simulink model "task8b_v23"  (R2023b)
settings: Solver=VariableStepAuto  StartTime=0.0  StopTime=10.0  RelTol=1e-3
values from neighbouring files (symbols this model uses):
  tInterval = [0 5]    [task7b2.m]    (also in task8b_setup.m = [0 10]; task9_visu.m = [0 10]; task9b_setup.m = [0 10])
undefined symbols (not defined in the file or in its folder): eul2tform, trvec2tform
libraries: robotcorelib x5, robotmaniplib x1
settings Model: Creator=Nico  LastModifiedBy=Nico
settings DebuggingCC: UnderSpecifiedDimensionMsg=warning
settings RTWCC: GPUComputeCapability=5.0

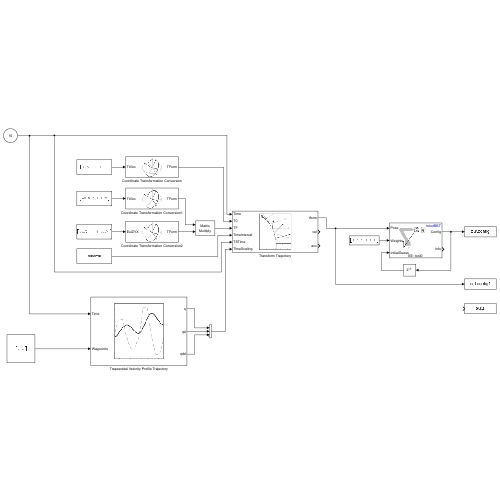
[thumbnail: Simulink's stored preview of the top-level diagram]
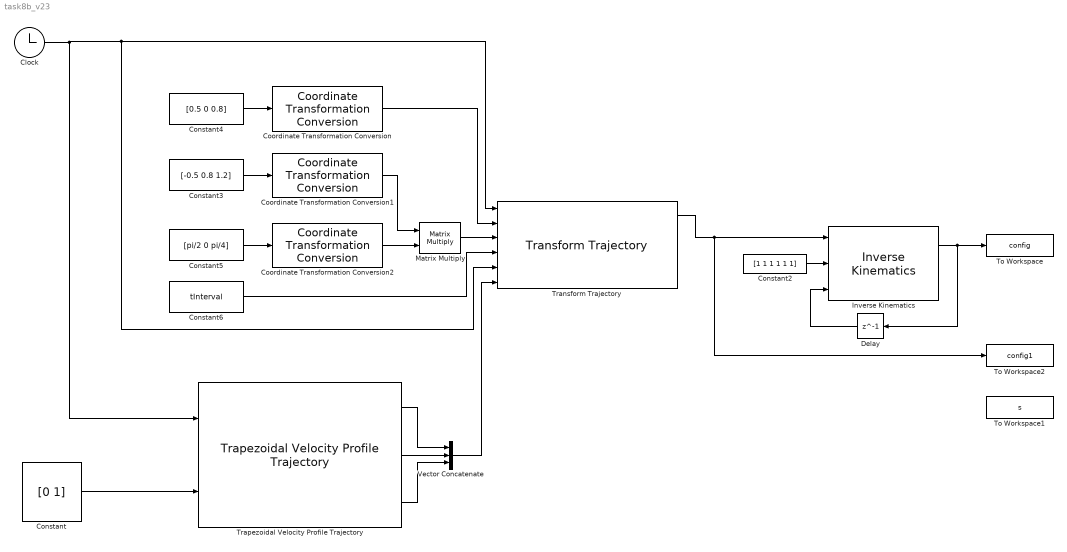
== system task8b_v23 ==
  Clock : Clock
  Constant : Constant  Value=[0 1]  VectorParams1D=off
  Constant2 : Constant  Value=[1 1 1 1 1 1]
  Constant3 : Constant  Value=[-0.5 0.8 1.2]
  Constant4 : Constant  Value=[0.5 0 0.8]
  Constant5 : Constant  Value=[pi/2 0 pi/4]
  Constant6 : Constant  Value=tInterval
  Coordinate Transformation Conversion : robotcorelib/Coordinate Transformation Conversion  InputRepresentation=Translation Vector  InputEulerSequence=ZYX  ShowTrVecInputPort=on  OutputRepresentation=Homogeneous Transformation  OutputEulerSequence=ZYX  ShowTrVecOutputPort=on  SimulateUsing=Interpreted execution
  Coordinate Transformation Conversion1 : robotcorelib/Coordinate Transformation Conversion  InputRepresentation=Translation Vector  InputEulerSequence=ZYX  ShowTrVecInputPort=on  OutputRepresentation=Homogeneous Transformation  OutputEulerSequence=ZYX  ShowTrVecOutputPort=off  SimulateUsing=Interpreted execution
  Coordinate Transformation Conversion2 : robotcorelib/Coordinate Transformation Conversion  InputRepresentation=Euler Angles  InputEulerSequence=ZYX  ShowTrVecInputPort=off  OutputRepresentation=Homogeneous Transformation  OutputEulerSequence=ZYX  ShowTrVecOutputPort=on  SimulateUsing=Interpreted execution
  Delay : Delay  DelayLength=1  InitialCondition=0
  Inverse Kinematics : robotmaniplib/Inverse Kinematics  RigidBodyTree=robotRBT  EndEffector=tool0  ShowInfo=on  SolverName=BFGS Gradient Projection  EnforceJointLimits=on  MaxIterations=1500  MaxTime=10  GradientTolerance=1e-7  SolutionTolerance=1e-6  StepTolerance=1e-14  ErrorChangeTolerance=1e-12  UseErrorDamping=on  DampingBias=0.0025  SimulateUsing=Interpreted execution
  Matrix Multiply : Product  Multiplication=Matrix(*)
  To Workspace : ToWorkspace  VariableName=config  SampleTime=-1
  To Workspace1 : ToWorkspace  VariableName=s  SampleTime=-1
  To Workspace2 : ToWorkspace  VariableName=config1  SampleTime=-1
  Transform Trajectory : robotcorelib/Transform Trajectory  WaypointSource=External  T0=trvec2tform( [ 1, 10, -1 ] )  TF=eul2tform( [ 0, pi, pi / 2 ] )  TimeInterval=[ 2, 3 ]  CustomTimeScaling=on  ParameterSource=External  TSTime=2:0.1:3  TimeScaling=[ 0:0.1:1; ones( 1, 11 ); zeros( 1, 11 ) ]  SimulateUsing=Interpreted execution
      settings: LibrarySourceBlock=robotutilslib/Transform Trajectory
  Trapezoidal Velocity Profile Trajectory : robotcorelib/Trapezoidal Velocity Profile Trajectory  WaypointSource=External  Waypoints=[ 0, -0.5, -1; 0, 0.5, 1 ]  NumParams=0  Parameter1=End Time  Parameter2=End Time  ParameterSource=External  PeakVelocity=[ 2; 2 ]  Acceleration=[ 1; 2 ]  EndTime=[ 1; 1 ]  AccelTime=[ 1; 2 ]  SimulateUsing=Code generation
  Vector Concatenate : Concatenate  NumInputs=3  Mode=Multidimensional array
  wires:
  Transform Trajectory/1 -> To Workspace2/1, Inverse Kinematics/1
  Inverse Kinematics/1 -> Delay/1, To Workspace/1
  Constant2/1 -> Inverse Kinematics/2
  Delay/1 -> Inverse Kinematics/3
  Clock/1 -> Trapezoidal Velocity Profile Trajectory/1, Transform Trajectory/1, Transform Trajectory/5
  Coordinate Transformation Conversion/1 -> Transform Trajectory/2
  Constant4/1 -> Coordinate Transformation Conversion/1
  Constant3/1 -> Coordinate Transformation Conversion1/1
  Constant5/1 -> Coordinate Transformation Conversion2/1
  Coordinate Transformation Conversion1/1 -> Matrix Multiply/1
  Coordinate Transformation Conversion2/1 -> Matrix Multiply/2
  Constant6/1 -> Transform Trajectory/4
  Matrix Multiply/1 -> Transform Trajectory/3
  Constant/1 -> Trapezoidal Velocity Profile Trajectory/2
  Vector Concatenate/1 -> Transform Trajectory/6
  Trapezoidal Velocity Profile Trajectory/1 -> Vector Concatenate/1
  Trapezoidal Velocity Profile Trajectory/2 -> Vector Concatenate/2
  Trapezoidal Velocity Profile Trajectory/3 -> Vector Concatenate/3
